simulink model "type2_PID"  (R2023b)
settings: Solver=ode1  StartTime=0.0  StopTime=15  FixedStep=0.01  RelTol=1e-3
libraries: slpidlib x4, simulink x1
settings Model: Creator=vanch  LastModifiedBy=vanch
settings DebuggingCC: UnderSpecifiedDimensionMsg=warning

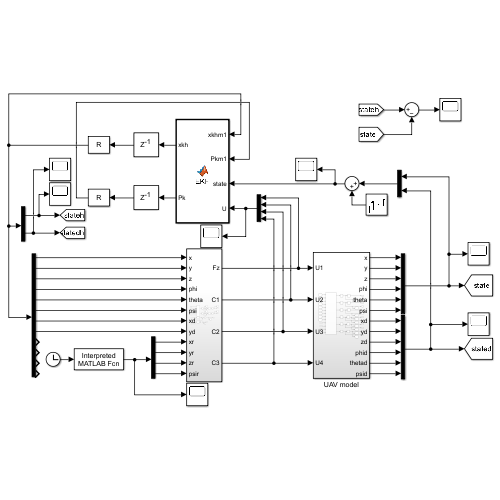
[thumbnail: Simulink's stored preview of the top-level diagram]
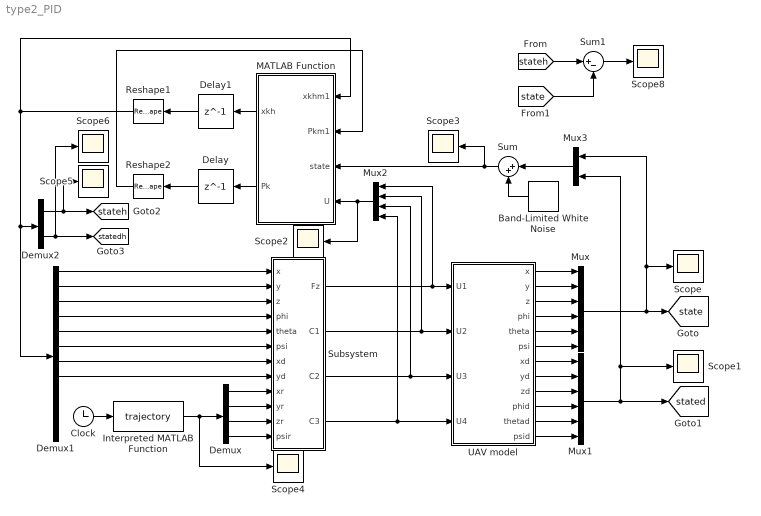
== system type2_PID ==
  Band-Limited White Noise : simulink/Sources/Band-Limited White Noise  Cov=1e-8  Ts=0.01  seed=[1535]
  Clock : Clock
  Delay : Delay  DelayLength=1  InitialCondition=(1e-3)*eye(12,12)
  Delay1 : Delay  DelayLength=1  InitialCondition=0.01
  Demux : Demux
  Demux1 : Demux  Outputs=12
  Demux2 : Demux  Outputs=2
  Interpreted MATLAB Function : MATLABFcn  MATLABFcn=trajectory  OutputDimensions=4
  MATLAB Function : MATLAB Function  TreatAsAtomicUnit=on
  Mux : Mux  Inputs=6
  Mux1 : Mux  Inputs=6
  Mux2 : Mux
  Mux3 : Mux  Inputs=2
  Reshape1 : Reshape  OutputDimensionality=Customize  OutputDimensions=[12,1]
  Reshape2 : Reshape  OutputDimensionality=Customize  OutputDimensions=[12,12]
  Scope{,1..6,8} (8 alike) : Scope
  Subsystem : Subsystem
  Sum : Sum  Inputs=|++
  Sum1 : Sum  Inputs=|+-
  UAV model : Subsystem
  tag scope: state=global, stated=global, statedh=global, stateh=global
  wires:
  UAV model/1(x) -> Mux/1
  UAV model/2(y) -> Mux/2
  UAV model/3(z) -> Mux/3
  UAV model/4(phi) -> Mux/4
  UAV model/5(theta) -> Mux/5
  UAV model/6(psi) -> Mux/6
  UAV model/7(xd) -> Mux1/1
  UAV model/8(yd) -> Mux1/2
  UAV model/9(zd) -> Mux1/3
  UAV model/10(phid) -> Mux1/4
  UAV model/11(thetad) -> Mux1/5
  UAV model/12(psid) -> Mux1/6
  Demux1/1 -> Subsystem/1(x)
  Demux1/2 -> Subsystem/2(y)
  Demux1/3 -> Subsystem/3(z)
  Demux1/4 -> Subsystem/4(phi)
  Demux1/5 -> Subsystem/5(theta)
  Demux1/6 -> Subsystem/6(psi)
  Subsystem/1(Fz) -> Mux2/1, UAV model/1(U1)
  Mux3/1 -> Sum/1
  Reshape2/1 -> MATLAB Function/2(Pkm1)
  Band-Limited White Noise/1 -> Sum/2
  Delay/1 -> Reshape2/1
  MATLAB Function/1(xkh) -> Delay1/1
  Sum/1 -> Scope3/1, MATLAB Function/3(state)
  Delay1/1 -> Reshape1/1
  MATLAB Function/2(Pk) -> Delay/1
  Mux2/1 -> MATLAB Function/4(U), Scope2/1
  Subsystem/2(C1) -> Mux2/2, UAV model/2(U2)
  Subsystem/3(C2) -> Mux2/3, UAV model/3(U3)
  Reshape1/1 -> Demux2/1, Demux1/1, MATLAB Function/1(xkhm1)
  Subsystem/4(C3) -> Mux2/4, UAV model/4(U4)
  Mux1/1 -> Mux3/2, Scope1/1, [stated]
  Mux/1 -> Mux3/1, Scope/1, [state]
  Demux1/7 -> Subsystem/7(xd)
  Demux1/8 -> Subsystem/8(yd)
  Demux/1 -> Subsystem/9(xr)
  Demux/2 -> Subsystem/10(yr)
  Demux/3 -> Subsystem/11(zr)
  Demux/4 -> Subsystem/12(psir)
  Interpreted MATLAB Function/1 -> Scope4/1, Demux/1
  Clock/1 -> Interpreted MATLAB Function/1
  Demux2/1 -> [stateh], Scope5/1
  Demux2/2 -> Scope6/1, [statedh]
  Sum1/1 -> Scope8/1
  [stateh] -> Sum1/1
  [state] -> Sum1/2

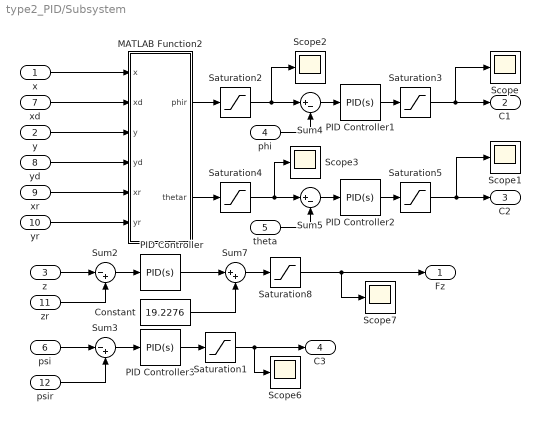
== system type2_PID/Subsystem ==
  x : Inport
  y : Inport  Port=2
  z : Inport  Port=3
  phi : Inport  Port=4
  theta : Inport  Port=5
  psi : Inport  Port=6
  xd : Inport  Port=7
  yd : Inport  Port=8
  xr : Inport  Port=9
  yr : Inport  Port=10
  zr : Inport  Port=11
  psir : Inport  Port=12
  Constant : Constant  Value=19.2276
  MATLAB Function2 : MATLAB Function  TreatAsAtomicUnit=on
  PID Controller : slpidlib/PID Controller  Controller=PID  Form=Parallel  TimeDomain=Continuous-time  UseExternalTs=off  SampleTime=-1  IntegratorMethod=Forward Euler  FilterMethod=Forward Euler  ControllerParametersSource=internal  P=10  I=0  UseKiTs=off  D=12  N=5  UseFilter=on  TunerSelectOption=Transfer Function Based (PID Tuner App)  InitialConditionSource=internal  InitialConditionForIntegrator=0  InitialConditionForFilter=0  DifferentiatorICPrevScaledInput=0  ExternalReset=none  TrackingMode=off  Kt=1  LimitOutput=off  SatLimitsSource=internal  UpperSaturationLimit=25  LowerSaturationLimit=0  LinearizeAsGain=on  AntiWindupMode=none  Kb=1  LimitIntegrator=off  UpperIntegratorSaturationLimit=inf  LowerIntegratorSaturationLimit=-inf  POutMin=[]  POutMax=[]  IOutMin=[]  IOutMax=[]  DOutMin=[]  DOutMax=[]  NOutMin=[]  NOutMax=[]  SumOutMin=[]  SumOutMax=[]  SaturationOutMin=[]  SaturationOutMax=[]  PParamMin=[]  PParamMax=[]  IParamMin=[]  IParamMax=[]  DParamMin=[]  DParamMax=[]  NParamMin=[]  NParamMax=[]  KbParamMin=[]  KbParamMax=[]  KtParamMin=[]  KtParamMax=[]  KbOutMin=[]  KbOutMax=[]  KtOutMin=[]  KtOutMax=[]  IntegratorOutMin=[]  IntegratorOutMax=[]  FilterOutMin=[]  FilterOutMax=[]  SumI1OutMin=[]  SumI1OutMax=[]  SumI2OutMin=[]  SumI2OutMax=[]  SumI3OutMin=[]  SumI3OutMax=[]  SumI4OutMin=[]  SumI4OutMax=[]  SumDOutMin=[]  SumDOutMax=[]  DifferentiatorOutMin=[]  DifferentiatorOutMax=[]  FilterDiffOutCoefMin=[]  FilterDiffOutCoefMax=[]  ReciprocalOutMin=[]  ReciprocalOutMax=[]  SumDenOutMin=[]  SumDenOutMax=[]  SumNumOutMin=[]  SumNumOutMax=[]  DivideOutMin=[]  DivideOutMax=[]  UdiffTsProdOutMin=[]  UdiffTsProdOutMax=[]  NTsProdOutMin=[]  NTsProdOutMax=[]  UintegralTsProdOutMin=[]  UintegralTsProdOutMax=[]  UngainTsProdOutMin=[]  UngainTsProdOutMax=[]  ClampingZeroOutDataTypeStr=Inherit: Inherit via back propagation  ClampingZeroOutMin=[]  ClampingZeroOutMax=[]  FilterDenConstantOutDataTypeStr=Inherit: Inherit via back propagation  FilterDenConstantOutMin=[]  FilterDenConstantOutMax=[]  PCopyOutDataTypeStr=Inherit: Inherit via back propagation  PCopyOutMin=[]  PCopyOutMax=[]  NCopyOutDataTypeStr=Inherit: Inherit via back propagation  NCopyOutMin=[]  NCopyOutMax=[]  IntegratorContinuousStateAttributes=''  IntegratorStateMustResolveToSignalObject=off  IntegratorRTWStateStorageClass=Auto  FilterContinuousStateAttributes=''  FilterStateMustResolveToSignalObject=off  FilterRTWStateStorageClass=Auto  ParallelPVariant=InternalParameters  IdealPVariant=Disabled  IVariant=InternalParameters  DVariant=InternalParameters  IntegratorVariant=Continuous  SatVariant=Disabled  AWVariant=Passthrough  PCopyVariant=Disabled  TRVariant=Disabled  FdbkBlocksVariant=Forward  IdealPFdbkVariant=Disabled  SatFdbkVariant=Disabled  DerivativeFilterVariant=ContFilter  NVariant=InternalParameters  NCopyVariant=Disabled  FilterICVariant=InternalICsFilter  IntegratorICVariant=InternalICs  ExternalResetVariant=Disabled  TRSumVariant=Passthrough  SumFdbkVariant=Disabled  SumVariant=Sum_PID  TsampFilterVariant=InternalTs  TsampNgainVariant=Passthrough  TsampIntegralVariant=Disabled_SignalSpec  ExternalSaturationOutDataTypeStr=Inherit: Same as second input
  PID Controller1 : slpidlib/PID Controller  Controller=PID  Form=Parallel  TimeDomain=Continuous-time  UseExternalTs=off  SampleTime=-1  IntegratorMethod=Forward Euler  FilterMethod=Forward Euler  ControllerParametersSource=internal  P=0.06  I=0  UseKiTs=off  D=0.04  N=20  UseFilter=on  TunerSelectOption=Transfer Function Based (PID Tuner App)  InitialConditionSource=internal  InitialConditionForIntegrator=0  InitialConditionForFilter=0  DifferentiatorICPrevScaledInput=0  ExternalReset=none  TrackingMode=off  Kt=1  LimitOutput=off  SatLimitsSource=internal  UpperSaturationLimit=0.05  LowerSaturationLimit=-0.05  LinearizeAsGain=on  AntiWindupMode=none  Kb=1  LimitIntegrator=off  UpperIntegratorSaturationLimit=inf  LowerIntegratorSaturationLimit=-inf  POutMin=[]  POutMax=[]  IOutMin=[]  IOutMax=[]  DOutMin=[]  DOutMax=[]  NOutMin=[]  NOutMax=[]  SumOutMin=[]  SumOutMax=[]  SaturationOutMin=[]  SaturationOutMax=[]  PParamMin=[]  PParamMax=[]  IParamMin=[]  IParamMax=[]  DParamMin=[]  DParamMax=[]  NParamMin=[]  NParamMax=[]  KbParamMin=[]  KbParamMax=[]  KtParamMin=[]  KtParamMax=[]  KbOutMin=[]  KbOutMax=[]  KtOutMin=[]  KtOutMax=[]  IntegratorOutMin=[]  IntegratorOutMax=[]  FilterOutMin=[]  FilterOutMax=[]  SumI1OutMin=[]  SumI1OutMax=[]  SumI2OutMin=[]  SumI2OutMax=[]  SumI3OutMin=[]  SumI3OutMax=[]  SumI4OutMin=[]  SumI4OutMax=[]  SumDOutMin=[]  SumDOutMax=[]  DifferentiatorOutMin=[]  DifferentiatorOutMax=[]  FilterDiffOutCoefMin=[]  FilterDiffOutCoefMax=[]  ReciprocalOutMin=[]  ReciprocalOutMax=[]  SumDenOutMin=[]  SumDenOutMax=[]  SumNumOutMin=[]  SumNumOutMax=[]  DivideOutMin=[]  DivideOutMax=[]  UdiffTsProdOutMin=[]  UdiffTsProdOutMax=[]  NTsProdOutMin=[]  NTsProdOutMax=[]  UintegralTsProdOutMin=[]  UintegralTsProdOutMax=[]  UngainTsProdOutMin=[]  UngainTsProdOutMax=[]  ClampingZeroOutDataTypeStr=Inherit: Inherit via back propagation  ClampingZeroOutMin=[]  ClampingZeroOutMax=[]  FilterDenConstantOutDataTypeStr=Inherit: Inherit via back propagation  FilterDenConstantOutMin=[]  FilterDenConstantOutMax=[]  PCopyOutDataTypeStr=Inherit: Inherit via back propagation  PCopyOutMin=[]  PCopyOutMax=[]  NCopyOutDataTypeStr=Inherit: Inherit via back propagation  NCopyOutMin=[]  NCopyOutMax=[]  IntegratorContinuousStateAttributes=''  IntegratorStateMustResolveToSignalObject=off  IntegratorRTWStateStorageClass=Auto  FilterContinuousStateAttributes=''  FilterStateMustResolveToSignalObject=off  FilterRTWStateStorageClass=Auto  ParallelPVariant=InternalParameters  IdealPVariant=Disabled  IVariant=InternalParameters  DVariant=InternalParameters  IntegratorVariant=Continuous  SatVariant=Disabled  AWVariant=Passthrough  PCopyVariant=Disabled  TRVariant=Disabled  FdbkBlocksVariant=Forward  IdealPFdbkVariant=Disabled  SatFdbkVariant=Disabled  DerivativeFilterVariant=ContFilter  NVariant=InternalParameters  NCopyVariant=Disabled  FilterICVariant=InternalICsFilter  IntegratorICVariant=InternalICs  ExternalResetVariant=Disabled  TRSumVariant=Passthrough  SumFdbkVariant=Disabled  SumVariant=Sum_PID  TsampFilterVariant=InternalTs  TsampNgainVariant=Passthrough  TsampIntegralVariant=Disabled_SignalSpec  ExternalSaturationOutDataTypeStr=Inherit: Same as second input
  PID Controller2 : slpidlib/PID Controller  Controller=PID  Form=Parallel  TimeDomain=Continuous-time  UseExternalTs=off  SampleTime=-1  IntegratorMethod=Forward Euler  FilterMethod=Forward Euler  ControllerParametersSource=internal  P=0.06  I=0  UseKiTs=off  D=0.04  N=20  UseFilter=on  TunerSelectOption=Transfer Function Based (PID Tuner App)  InitialConditionSource=internal  InitialConditionForIntegrator=0  InitialConditionForFilter=0  DifferentiatorICPrevScaledInput=0  ExternalReset=none  TrackingMode=off  Kt=1  LimitOutput=off  SatLimitsSource=internal  UpperSaturationLimit=0.05  LowerSaturationLimit=-0.05  LinearizeAsGain=on  AntiWindupMode=none  Kb=1  LimitIntegrator=off  UpperIntegratorSaturationLimit=inf  LowerIntegratorSaturationLimit=-inf  POutMin=[]  POutMax=[]  IOutMin=[]  IOutMax=[]  DOutMin=[]  DOutMax=[]  NOutMin=[]  NOutMax=[]  SumOutMin=[]  SumOutMax=[]  SaturationOutMin=[]  SaturationOutMax=[]  PParamMin=[]  PParamMax=[]  IParamMin=[]  IParamMax=[]  DParamMin=[]  DParamMax=[]  NParamMin=[]  NParamMax=[]  KbParamMin=[]  KbParamMax=[]  KtParamMin=[]  KtParamMax=[]  KbOutMin=[]  KbOutMax=[]  KtOutMin=[]  KtOutMax=[]  IntegratorOutMin=[]  IntegratorOutMax=[]  FilterOutMin=[]  FilterOutMax=[]  SumI1OutMin=[]  SumI1OutMax=[]  SumI2OutMin=[]  SumI2OutMax=[]  SumI3OutMin=[]  SumI3OutMax=[]  SumI4OutMin=[]  SumI4OutMax=[]  SumDOutMin=[]  SumDOutMax=[]  DifferentiatorOutMin=[]  DifferentiatorOutMax=[]  FilterDiffOutCoefMin=[]  FilterDiffOutCoefMax=[]  ReciprocalOutMin=[]  ReciprocalOutMax=[]  SumDenOutMin=[]  SumDenOutMax=[]  SumNumOutMin=[]  SumNumOutMax=[]  DivideOutMin=[]  DivideOutMax=[]  UdiffTsProdOutMin=[]  UdiffTsProdOutMax=[]  NTsProdOutMin=[]  NTsProdOutMax=[]  UintegralTsProdOutMin=[]  UintegralTsProdOutMax=[]  UngainTsProdOutMin=[]  UngainTsProdOutMax=[]  ClampingZeroOutDataTypeStr=Inherit: Inherit via back propagation  ClampingZeroOutMin=[]  ClampingZeroOutMax=[]  FilterDenConstantOutDataTypeStr=Inherit: Inherit via back propagation  FilterDenConstantOutMin=[]  FilterDenConstantOutMax=[]  PCopyOutDataTypeStr=Inherit: Inherit via back propagation  PCopyOutMin=[]  PCopyOutMax=[]  NCopyOutDataTypeStr=Inherit: Inherit via back propagation  NCopyOutMin=[]  NCopyOutMax=[]  IntegratorContinuousStateAttributes=''  IntegratorStateMustResolveToSignalObject=off  IntegratorRTWStateStorageClass=Auto  FilterContinuousStateAttributes=''  FilterStateMustResolveToSignalObject=off  FilterRTWStateStorageClass=Auto  ParallelPVariant=InternalParameters  IdealPVariant=Disabled  IVariant=InternalParameters  DVariant=InternalParameters  IntegratorVariant=Continuous  SatVariant=Disabled  AWVariant=Passthrough  PCopyVariant=Disabled  TRVariant=Disabled  FdbkBlocksVariant=Forward  IdealPFdbkVariant=Disabled  SatFdbkVariant=Disabled  DerivativeFilterVariant=ContFilter  NVariant=InternalParameters  NCopyVariant=Disabled  FilterICVariant=InternalICsFilter  IntegratorICVariant=InternalICs  ExternalResetVariant=Disabled  TRSumVariant=Passthrough  SumFdbkVariant=Disabled  SumVariant=Sum_PID  TsampFilterVariant=InternalTs  TsampNgainVariant=Passthrough  TsampIntegralVariant=Disabled_SignalSpec  ExternalSaturationOutDataTypeStr=Inherit: Same as second input
  PID Controller3 : slpidlib/PID Controller  Controller=PID  Form=Parallel  TimeDomain=Continuous-time  UseExternalTs=off  SampleTime=-1  IntegratorMethod=Forward Euler  FilterMethod=Forward Euler  ControllerParametersSource=internal  P=0.04  I=0  UseKiTs=off  D=0.03  N=100  UseFilter=on  TunerSelectOption=Transfer Function Based (PID Tuner App)  InitialConditionSource=internal  InitialConditionForIntegrator=0  InitialConditionForFilter=0  DifferentiatorICPrevScaledInput=0  ExternalReset=none  TrackingMode=off  Kt=1  LimitOutput=off  SatLimitsSource=internal  UpperSaturationLimit=0.05  LowerSaturationLimit=-0.05  LinearizeAsGain=on  AntiWindupMode=none  Kb=1  LimitIntegrator=off  UpperIntegratorSaturationLimit=inf  LowerIntegratorSaturationLimit=-inf  POutMin=[]  POutMax=[]  IOutMin=[]  IOutMax=[]  DOutMin=[]  DOutMax=[]  NOutMin=[]  NOutMax=[]  SumOutMin=[]  SumOutMax=[]  SaturationOutMin=[]  SaturationOutMax=[]  PParamMin=[]  PParamMax=[]  IParamMin=[]  IParamMax=[]  DParamMin=[]  DParamMax=[]  NParamMin=[]  NParamMax=[]  KbParamMin=[]  KbParamMax=[]  KtParamMin=[]  KtParamMax=[]  KbOutMin=[]  KbOutMax=[]  KtOutMin=[]  KtOutMax=[]  IntegratorOutMin=[]  IntegratorOutMax=[]  FilterOutMin=[]  FilterOutMax=[]  SumI1OutMin=[]  SumI1OutMax=[]  SumI2OutMin=[]  SumI2OutMax=[]  SumI3OutMin=[]  SumI3OutMax=[]  SumI4OutMin=[]  SumI4OutMax=[]  SumDOutMin=[]  SumDOutMax=[]  DifferentiatorOutMin=[]  DifferentiatorOutMax=[]  FilterDiffOutCoefMin=[]  FilterDiffOutCoefMax=[]  ReciprocalOutMin=[]  ReciprocalOutMax=[]  SumDenOutMin=[]  SumDenOutMax=[]  SumNumOutMin=[]  SumNumOutMax=[]  DivideOutMin=[]  DivideOutMax=[]  UdiffTsProdOutMin=[]  UdiffTsProdOutMax=[]  NTsProdOutMin=[]  NTsProdOutMax=[]  UintegralTsProdOutMin=[]  UintegralTsProdOutMax=[]  UngainTsProdOutMin=[]  UngainTsProdOutMax=[]  ClampingZeroOutDataTypeStr=Inherit: Inherit via back propagation  ClampingZeroOutMin=[]  ClampingZeroOutMax=[]  FilterDenConstantOutDataTypeStr=Inherit: Inherit via back propagation  FilterDenConstantOutMin=[]  FilterDenConstantOutMax=[]  PCopyOutDataTypeStr=Inherit: Inherit via back propagation  PCopyOutMin=[]  PCopyOutMax=[]  NCopyOutDataTypeStr=Inherit: Inherit via back propagation  NCopyOutMin=[]  NCopyOutMax=[]  IntegratorContinuousStateAttributes=''  IntegratorStateMustResolveToSignalObject=off  IntegratorRTWStateStorageClass=Auto  FilterContinuousStateAttributes=''  FilterStateMustResolveToSignalObject=off  FilterRTWStateStorageClass=Auto  ParallelPVariant=InternalParameters  IdealPVariant=Disabled  IVariant=InternalParameters  DVariant=InternalParameters  IntegratorVariant=Continuous  SatVariant=Disabled  AWVariant=Passthrough  PCopyVariant=Disabled  TRVariant=Disabled  FdbkBlocksVariant=Forward  IdealPFdbkVariant=Disabled  SatFdbkVariant=Disabled  DerivativeFilterVariant=ContFilter  NVariant=InternalParameters  NCopyVariant=Disabled  FilterICVariant=InternalICsFilter  IntegratorICVariant=InternalICs  ExternalResetVariant=Disabled  TRSumVariant=Passthrough  SumFdbkVariant=Disabled  SumVariant=Sum_PID  TsampFilterVariant=InternalTs  TsampNgainVariant=Passthrough  TsampIntegralVariant=Disabled_SignalSpec  ExternalSaturationOutDataTypeStr=Inherit: Same as second input
  Saturation1 : Saturate  UpperLimit=0.01  LowerLimit=-0.01
  Saturation2 : Saturate  UpperLimit=0.2  LowerLimit=-0.2
  Saturation3 : Saturate  UpperLimit=0.01  LowerLimit=-0.01
  Saturation4 : Saturate  UpperLimit=0.2  LowerLimit=-0.2
  Saturation5 : Saturate  UpperLimit=0.01  LowerLimit=-0.01
  Saturation8 : Saturate  UpperLimit=50  LowerLimit=0
  Scope{,1..3,6..7} (6 alike) : Scope
  Sum2 : Sum  Inputs=|-+
  Sum3 : Sum  Inputs=|-+
  Sum4 : Sum  Inputs=|+-
  Sum5 : Sum  Inputs=|+-
  Sum7 : Sum  Inputs=|++
  Fz : Outport
  C1 : Outport  Port=2
  C2 : Outport  Port=3
  C3 : Outport  Port=4
  wires:
  z/1 -> Sum2/1
  Sum2/1 -> PID Controller/1
  psi/1 -> Sum3/1
  Sum3/1 -> PID Controller3/1
  x/1 -> MATLAB Function2/1(x)
  y/1 -> MATLAB Function2/3(y)
  PID Controller3/1 -> Saturation1/1
  PID Controller/1 -> Sum7/1
  Sum7/1 -> Saturation8/1
  Constant/1 -> Sum7/2
  Saturation8/1 -> Fz/1, Scope7/1
  Saturation1/1 -> C3/1, Scope6/1
  PID Controller1/1 -> Saturation3/1
  Sum4/1 -> PID Controller1/1
  PID Controller2/1 -> Saturation5/1
  Saturation3/1 -> C1/1, Scope/1
  Sum5/1 -> PID Controller2/1
  MATLAB Function2/1(phir) -> Saturation2/1
  MATLAB Function2/2(thetar) -> Saturation4/1
  Saturation5/1 -> C2/1, Scope1/1
  phi/1 -> Sum4/2
  theta/1 -> Sum5/2
  xd/1 -> MATLAB Function2/2(xd)
  yd/1 -> MATLAB Function2/4(yd)
  xr/1 -> MATLAB Function2/5(xr)
  yr/1 -> MATLAB Function2/6(yr)
  zr/1 -> Sum2/2
  psir/1 -> Sum3/2
  Saturation2/1 -> Sum4/1, Scope2/1
  Saturation4/1 -> Sum5/1, Scope3/1

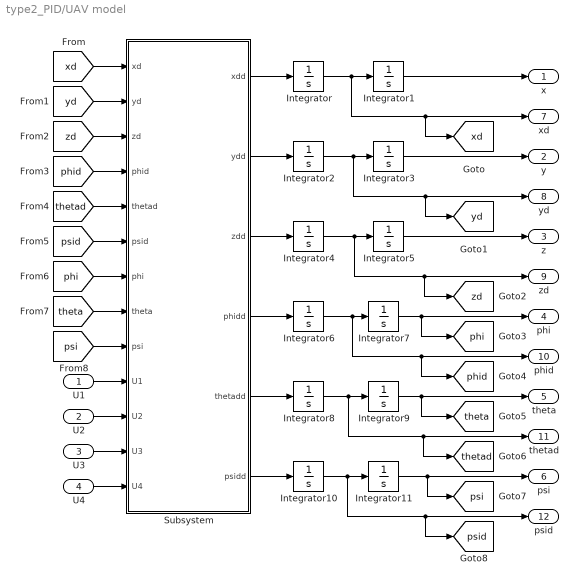
== system type2_PID/UAV model ==
  U1 : Inport
  U2 : Inport  Port=2
  U3 : Inport  Port=3
  U4 : Inport  Port=4
  Integrator{,1..4,6..11} (11 alike) : Integrator  InitialCondition=0.01
  Integrator5 : Integrator  InitialCondition=0.01  LimitOutput=on  LowerSaturationLimit=0
  Subsystem : Subsystem
  x : Outport
  y : Outport  Port=2
  z : Outport  Port=3
  phi : Outport  Port=4
  theta : Outport  Port=5
  psi : Outport  Port=6
  xd : Outport  Port=7
  yd : Outport  Port=8
  zd : Outport  Port=9
  phid : Outport  Port=10
  thetad : Outport  Port=11
  psid : Outport  Port=12
  tag scope: phi=global, phid=global, psi=global, psid=global, theta=global, thetad=global, xd=global, yd=global, zd=global
  wires:
  Integrator5/1 -> z/1
  Integrator6/1 -> phid/1, [phid], Integrator7/1
  Integrator1/1 -> x/1
  [psid] -> Subsystem/6(psid)
  Integrator2/1 -> yd/1, [yd], Integrator3/1
  Subsystem/3(zdd) -> Integrator4/1
  Subsystem/6(psidd) -> Integrator10/1
  Integrator3/1 -> y/1
  Integrator8/1 -> thetad/1, [thetad], Integrator9/1
  [theta] -> Subsystem/8(theta)
  Integrator/1 -> xd/1, [xd], Integrator1/1
  [thetad] -> Subsystem/5(thetad)
  [zd] -> Subsystem/3(zd)
  Subsystem/4(phidd) -> Integrator6/1
  Integrator9/1 -> theta/1, [theta]
  [phid] -> Subsystem/4(phid)
  Integrator10/1 -> psid/1, [psid], Integrator11/1
  Subsystem/2(ydd) -> Integrator2/1
  Integrator4/1 -> zd/1, [zd], Integrator5/1
  Subsystem/5(thetadd) -> Integrator8/1
  Subsystem/1(xdd) -> Integrator/1
  [yd] -> Subsystem/2(yd)
  [psi] -> Subsystem/9(psi)
  Integrator11/1 -> psi/1, [psi]
  [xd] -> Subsystem/1(xd)
  [phi] -> Subsystem/7(phi)
  Integrator7/1 -> phi/1, [phi]
  U1/1 -> Subsystem/10(U1)
  U2/1 -> Subsystem/11(U2)
  U3/1 -> Subsystem/12(U3)
  U4/1 -> Subsystem/13(U4)

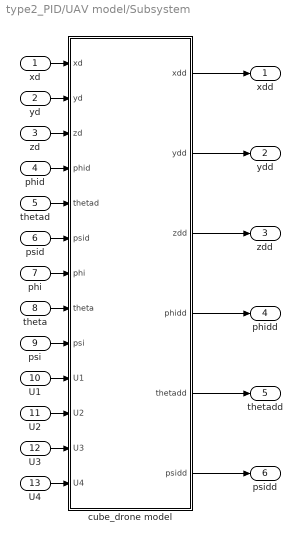
== system type2_PID/UAV model/Subsystem ==
  xd : Inport
  yd : Inport  Port=2
  zd : Inport  Port=3
  phid : Inport  Port=4
  thetad : Inport  Port=5
  psid : Inport  Port=6
  phi : Inport  Port=7
  theta : Inport  Port=8
  psi : Inport  Port=9
  U1 : Inport  Port=10
  U2 : Inport  Port=11
  U3 : Inport  Port=12
  U4 : Inport  Port=13
  cube_drone model : MATLAB Function  TreatAsAtomicUnit=on
  xdd : Outport
  ydd : Outport  Port=2
  zdd : Outport  Port=3
  phidd : Outport  Port=4
  thetadd : Outport  Port=5
  psidd : Outport  Port=6
  wires:
  U4/1 -> cube_drone model/13(U4)
  U1/1 -> cube_drone model/10(U1)
  U2/1 -> cube_drone model/11(U2)
  cube_drone model/2(ydd) -> ydd/1
  cube_drone model/4(phidd) -> phidd/1
  U3/1 -> cube_drone model/12(U3)
  cube_drone model/3(zdd) -> zdd/1
  cube_drone model/5(thetadd) -> thetadd/1
  psid/1 -> cube_drone model/6(psid)
  cube_drone model/6(psidd) -> psidd/1
  zd/1 -> cube_drone model/3(zd)
  yd/1 -> cube_drone model/2(yd)
  thetad/1 -> cube_drone model/5(thetad)
  phid/1 -> cube_drone model/4(phid)
  phi/1 -> cube_drone model/7(phi)
  cube_drone model/1(xdd) -> xdd/1
  xd/1 -> cube_drone model/1(xd)
  theta/1 -> cube_drone model/8(theta)
  psi/1 -> cube_drone model/9(psi)

== matlab function type2_PID/UAV model/Subsystem/cube_drone model ==
  data: xd input; xdd output; yd input; zd input; phid input; thetad input; psid input; phi input; theta input; psi input; U1 input; U2 input; U3 input; U4 input; ydd output; zdd output; phidd output; thetadd output; psidd output
function [xdd,ydd,zdd,phidd,thetadd,psidd] = fcn(xd,yd,zd,phid,thetad,psid,phi,theta,psi,U1,U2,U3,U4)
%cos,sin
cphi=cos(phi);
sphi=sin(phi);
ctheta=cos(theta);
stheta=sin(theta);
cpsi=cos(psi);
spsi=sin(psi);
%parameters
m=1.96;
g=9.81;
Kdx=0.00055670;
Kdy=0.00055670;
Kdz=0.0006354;
Ixx=0.00149;
Iyy=0.00153;
Izz=0.00532;
%motion equation
xdd=1/m*((spsi*sphi+cpsi*stheta*cphi)*U1-Kdx*xd);
ydd=1/m*((spsi*stheta*cphi-cpsi*sphi)*U1-Kdy*yd);
zdd=1/m*(ctheta*cphi*U1-Kdz*zd-m*g);
phidd=1/Ixx*(psid*thetad*(Iyy-Izz)+U2);
thetadd=1/Iyy*(psid*phid*(Izz-Ixx)+U3);
psidd=1/Izz*(phid*thetad*(Ixx-Iyy)+U4);
end

== matlab function type2_PID/Subsystem/MATLAB Function2 ==
  data: x input; phir output; xd input; thetar output; y input; yd input; xr input; yr input
function [phir,thetar] = fcn(x,xd,y,yd,xr,yr)
kpx=0.1;
kdx=0.15;
kpy=0.1;
kdy=0.15;
thetar=kpx*(xr-x)-kdx*xd;
phir=-kpy*(yr-y)+kdy*yd;
end

== matlab function type2_PID/MATLAB Function ==
  data: xkhm1 input; Pkm1 input; xkh output; state input; U input; Pk output
function [xkh,Pk] = EKF(xkhm1,Pkm1,state,U)
%parameters
dt=0.01;
Q=1e-6;
R=1e-5;
m=1.96;
g=9.81;
Kdx=0.00055670;
Kdy=0.00055670;
Kdz=0.0006354;
Ixx=0.00149;
Iyy=0.00153;
Izz=0.00532;
%states
x=xkhm1(1);
y=xkhm1(2);
z=xkhm1(3);
phi=xkhm1(4);
theta=xkhm1(5);
psi=xkhm1(6);
xd=xkhm1(7);
yd=xkhm1(8);
zd=xkhm1(9);
phid=xkhm1(10);
thetad=xkhm1(11);
psid=xkhm1(12);
%linearized
A=[0, 0, 0, 0, 0, 0, 1, 0, 0, 0, 0, 0;
   0, 0, 0, 0, 0, 0, 0, 1, 0, 0, 0, 0;
   0, 0, 0, 0, 0, 0, 0, 0, 1, 0, 0, 0;
   0, 0, 0, 0, 0, 0, 0, 0, 0, 1, 0, 0;
   0, 0, 0, 0, 0, 0, 0, 0, 0, 0, 1, 0;
   0, 0, 0, 0, 0, 0, 0, 0, 0, 0, 0, 1;
   0, 0, 0, 0, 0, 0, -Kdx/m, 0, 0, 0, 0, 0;
  0, 0, 0, 0, 0, 0, 0, -Kdy/m, 0, 0, 0, 0;
  0, 0, 0, 0, 0, 0, 0, 0, -Kdz/m, 0, 0, 0;
  0, 0, 0, 0, 0, 0, 0, 0, 0, 0, (psid*(Iyy - Izz))/Ixx, (thetad*(Iyy - Izz))/Ixx;
  0, 0, 0, 0, 0, 0, 0, 0, 0, -(psid*(Ixx - Izz))/Iyy, 0, -(phid*(Ixx - Izz))/Iyy;
  0, 0, 0, 0, 0, 0, 0, 0, 0, (thetad*(Ixx - Iyy))/Izz, (phid*(Ixx - Iyy))/Izz, 0];
B=[0, 0, 0, 0;
   0, 0, 0, 0;
   0, 0, 0, 0;
   0, 0, 0, 0;
   0, 0, 0, 0;
   0, 0, 0, 0;
   (sin(phi)*sin(psi) + cos(phi)*cos(psi)*sin(theta))/m, 0, 0, 0;
   -(cos(psi)*sin(phi) - cos(phi)*sin(psi)*sin(theta))/m, 0, 0, 0;
   (cos(phi)*cos(theta))/m, 0, 0 ,0;
   0, 1/Ixx, 0, 0;
   0, 0, 1/Iyy, 0;
   0, 0, 0, 1/Izz];
%Prediction
xkhm=xkhm1+A*xkhm1*dt+B*U*dt;
Pkm=A*Pkm1*A'+Q*eye(12);
%update
Kk=(Pkm*eye(12))/(eye(12)*Pkm*eye(12)+R*eye(12));
xkh=xkhm+Kk*(state-eye(12)*xkhm);
Pk=(eye(12)-Kk*eye*(12))*Pkm;
end
